simulink model "comparison_simulate_Hinf"  (R2015a)
settings: Solver=ode14x  StartTime=0.0  StopTime=10  FixedStep=1e-4  RelTol=1e-3
values from neighbouring files (symbols this model uses):
  A = [-209.443458109 -450.728478794 0 0 0 0 450.728478794 -209.443458109 0 0 0 0 ... (36 elements, 6x6)]    [comparison.mat]
  AC = [-33660.7984807 29637.8330782 3046.26276086 1989.6816824 595.970985765 1727.63504419 0 0 0 0 0 0 ... (400 elements, 20x20)]    [AC.mat]    (also in h2hinf.m = Kmix.A; hinf.m = K3.A)
  B = [-9.64474367822  2.65660382188; -7.76311006326  -5.61613187293; -0.117927290005  0.0527206875641; 0.215603654719  -0.128623447556; 0.0737096142171  0.0391127484963; -0.0970049785583  -0.0786358112919]    [comparison.mat]
  BC = [23360.0818714 -21011.7426002 -2127.29641138 -1389.45423788 -416.184367151 -1206.45923159 0 0 0 0 0 0 ... (20 elements, 20x1)]    [BC.mat]    (also in h2hinf.m = Kmix.B; hinf.m = K3.B)
  C = [1.88477251669 -1.14284793707 5.77230310808 47.9525873536 -5.11774457916 -49.0010462763]    [comparison.mat]
  CC = [0 0 0 0 0 0 0 0 0 0 0 0 ... (40 elements, 2x20)]    [CC.mat]    (also in h2hinf.m = Kmix.C; hinf.m = K3.C)
  DC = [0 0]    [DC.mat]    (also in h2hinf.m = Kmix.D; hinf.m = K3.D)
  H = [9.64474367822 7.76311006326 0.117927290005 -0.215603654719 -0.0737096142171 0.0970049785583]    [comparison.mat]
  K1 = [2.2796711846  1.62190033935  -10.6282516318  -1.4108556961  -12.4808932363  26.7941597177; 0.146705446363  -9.20812525479  8.2724414747  30.8052765889  17.6744281041  -4.60573511505]    [comparison.mat]
  K2 = [7.68340364795  3.76895934778  4.7809593416  1.0105906737  4.39829283468  -9.14553212992; -11.324326837  11.7994850376  -4.15081128654  -16.3715631545  -6.63659637257  1.48616499821]    [comparison.mat]
  L1 = [25.9427258674 3.21915313057 0.189903086471 -0.425157992773 0.204783234732 0.30836256894]    [comparison.mat]
  L2 = [-17.8178024007 12.2869558648 -0.241266463594 0.355791079936 -0.00240455397922 -0.130577661056]    [comparison.mat]
settings Model: Creator=p4wp4w  LastModifiedBy=p4wp4w

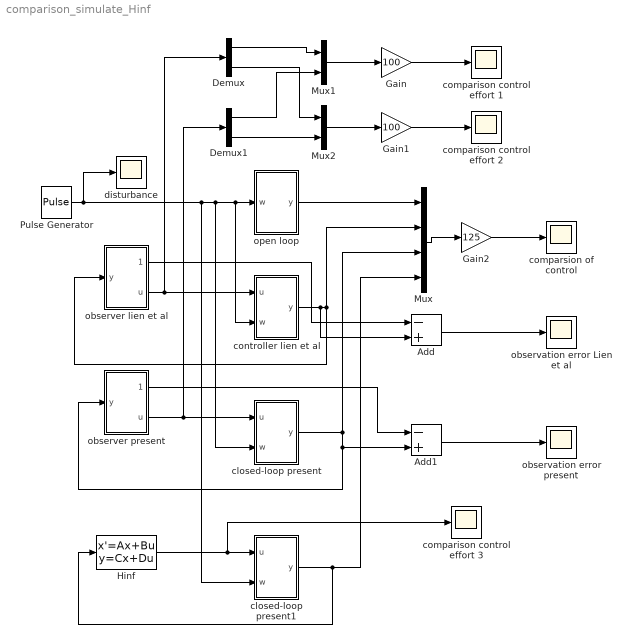
== system comparison_simulate_Hinf ==
  Add : Sum  Inputs=-+
  Add1 : Sum  Inputs=-+
  Demux : Demux  Outputs=2
  Demux1 : Demux  Outputs=2
  Gain : Gain  Gain=100
  Gain1 : Gain  Gain=100
  Gain2 : Gain  Gain=125
  Hinf : StateSpace  A=AC  B=BC  C=CC  D=DC  X0=0
  Mux : Mux
  Mux1 : Mux  Inputs=2
  Mux2 : Mux  Inputs=2
  Pulse Generator : DiscretePulseGenerator  PulseType=Time based  Amplitude=10  Period=5  PulseWidth=50
  closed-loop present : Subsystem
  closed-loop present1 : Subsystem
  comparison control effort 1 : Scope
      settings: SaveName=effort1
  comparison control effort 2 : Scope
      settings: SaveName=effort2
  comparison control effort 3 : Scope
      settings: SaveName=effort
  comparsion of control : Scope
      settings: YMin=-100  YMax=75  SaveName=controlleduncontrolled
  controller lien et al : Subsystem
  disturbance : Scope
      settings: SaveName=disturbance
  observation error Lien et al : Scope
      settings: SaveName=observation_error_Lien
  observation error present : Scope
      settings: SaveName=observation_error_present
  observer lien et al : Subsystem
  observer present : Subsystem
  open loop : Subsystem
  wires:
  controller lien et al/1(y) -> Add/2, Mux/2, observer lien et al/1(y)
  observer lien et al/2(u) -> Demux/1, controller lien et al/1(u)
  Pulse Generator/1 -> disturbance/1, closed-loop present1/2(w), closed-loop present/2(w), controller lien et al/2(w), open loop/1(w)
  observer present/2(u) -> Demux1/1, closed-loop present/1(u)
  closed-loop present/1(y) -> Add1/2, observer present/1(y), Mux/3
  open loop/1(y) -> Mux/1
  Mux/1 -> Gain2/1
  observer lien et al/1(yhat) -> Add/1
  observer present/1(yhat) -> Add1/1
  Mux1/1 -> Gain/1
  Gain/1 -> comparison control effort 1/1
  Mux2/1 -> Gain1/1
  Gain1/1 -> comparison control effort 2/1
  Demux1/1 -> Mux1/2
  Demux/1 -> Mux1/1
  Demux/2 -> Mux2/1
  Demux1/2 -> Mux2/2
  Gain2/1 -> comparsion of control/1
  Add/1 -> observation error Lien et al/1
  Add1/1 -> observation error present/1
  Hinf/1 -> comparison control effort 3/1, closed-loop present1/1(u)
  closed-loop present1/1(y) -> Mux/4, Hinf/1

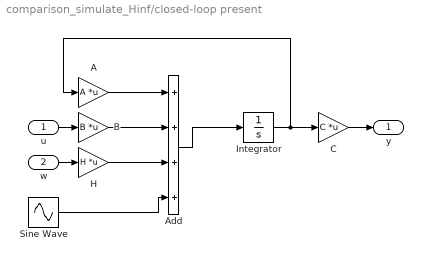
== system comparison_simulate_Hinf/closed-loop present ==
  u : Inport
  w : Inport  Port=2
  A : Gain  Gain=A  Multiplication=Matrix(K*u)
  Add : Sum  Inputs=++++
  B : Gain  Gain=B  Multiplication=Matrix(K*u)
  C : Gain  Gain=C  Multiplication=Matrix(K*u)
  H : Gain  Gain=H  Multiplication=Matrix(K*u)
  Integrator : Integrator
  Sine Wave : Sin  Amplitude=0.01  Frequency=14  SampleTime=0
  y : Outport
  wires:
  C/1 -> y/1
  u/1 -> B/1
  w/1 -> H/1
  H/1 -> Add/3
  Integrator/1 -> A/1, C/1
  A/1 -> Add/1
  B/1 -> Add/2
  Add/1 -> Integrator/1
  Sine Wave/1 -> Add/4

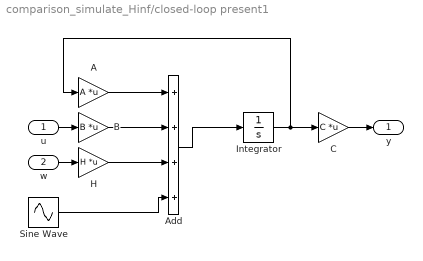
== system comparison_simulate_Hinf/closed-loop present1 ==
  u : Inport
  w : Inport  Port=2
  A : Gain  Gain=A  Multiplication=Matrix(K*u)
  Add : Sum  Inputs=++++
  B : Gain  Gain=B  Multiplication=Matrix(K*u)
  C : Gain  Gain=C  Multiplication=Matrix(K*u)
  H : Gain  Gain=H  Multiplication=Matrix(K*u)
  Integrator : Integrator
  Sine Wave : Sin  Amplitude=0.01  Frequency=14  SampleTime=0
  y : Outport
  wires:
  Sine Wave/1 -> Add/4
  Add/1 -> Integrator/1
  B/1 -> Add/2
  A/1 -> Add/1
  Integrator/1 -> C/1, A/1
  H/1 -> Add/3
  w/1 -> H/1
  u/1 -> B/1
  C/1 -> y/1

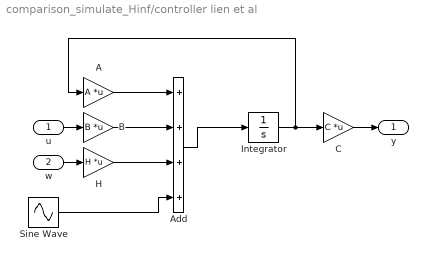
== system comparison_simulate_Hinf/controller lien et al ==
  u : Inport
  w : Inport  Port=2
  A : Gain  Gain=A  Multiplication=Matrix(K*u)
  Add : Sum  Inputs=++++
  B : Gain  Gain=B  Multiplication=Matrix(K*u)
  C : Gain  Gain=C  Multiplication=Matrix(K*u)
  H : Gain  Gain=H  Multiplication=Matrix(K*u)
  Integrator : Integrator
  Sine Wave : Sin  Amplitude=0.01  Frequency=14  SampleTime=0
  y : Outport
  wires:
  Add/1 -> Integrator/1
  B/1 -> Add/2
  A/1 -> Add/1
  Integrator/1 -> C/1, A/1
  H/1 -> Add/3
  w/1 -> H/1
  u/1 -> B/1
  C/1 -> y/1
  Sine Wave/1 -> Add/4

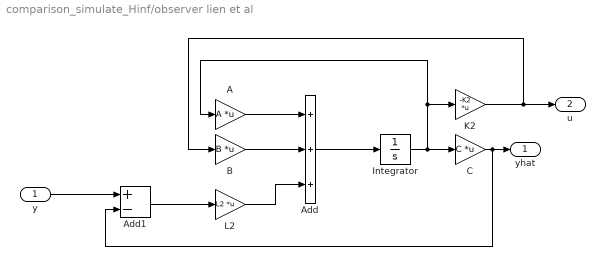
== system comparison_simulate_Hinf/observer lien et al ==
  y : Inport
  A : Gain  Gain=A  Multiplication=Matrix(K*u)
  Add : Sum  Inputs=+++
  Add1 : Sum  Inputs=+-
  B : Gain  Gain=B  Multiplication=Matrix(K*u)
  C : Gain  Gain=C  Multiplication=Matrix(K*u)
  Integrator : Integrator
  K2 : Gain  Gain=-K2  Multiplication=Matrix(K*u)
  L2 : Gain  Gain=L2  Multiplication=Matrix(K*u)
  yhat : Outport
  u : Outport  Port=2
  wires:
  C/1 -> Add1/2, yhat/1
  K2/1 -> B/1, u/1
  Integrator/1 -> K2/1, A/1, C/1
  A/1 -> Add/1
  B/1 -> Add/2
  Add/1 -> Integrator/1
  L2/1 -> Add/3
  Add1/1 -> L2/1
  y/1 -> Add1/1

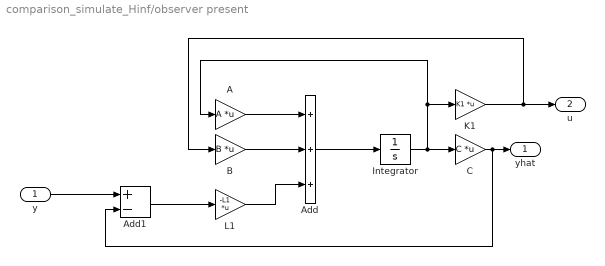
== system comparison_simulate_Hinf/observer present ==
  y : Inport
  A : Gain  Gain=A  Multiplication=Matrix(K*u)
  Add : Sum  Inputs=+++
  Add1 : Sum  Inputs=+-
  B : Gain  Gain=B  Multiplication=Matrix(K*u)
  C : Gain  Gain=C  Multiplication=Matrix(K*u)
  Integrator : Integrator
  K1 : Gain  Gain=K1  Multiplication=Matrix(K*u)
  L1 : Gain  Gain=-L1  Multiplication=Matrix(K*u)
  yhat : Outport
  u : Outport  Port=2
  wires:
  y/1 -> Add1/1
  Add1/1 -> L1/1
  L1/1 -> Add/3
  Add/1 -> Integrator/1
  B/1 -> Add/2
  A/1 -> Add/1
  Integrator/1 -> C/1, A/1, K1/1
  K1/1 -> u/1, B/1
  C/1 -> yhat/1, Add1/2

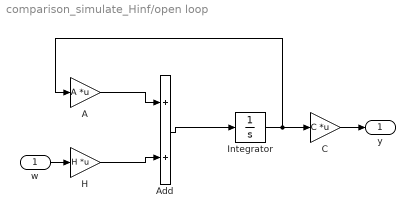
== system comparison_simulate_Hinf/open loop ==
  w : Inport
  A : Gain  Gain=A  Multiplication=Matrix(K*u)
  Add : Sum
  C : Gain  Gain=C  Multiplication=Matrix(K*u)
  H : Gain  Gain=H  Multiplication=Matrix(K*u)
  Integrator : Integrator
  y : Outport
  wires:
  C/1 -> y/1
  w/1 -> H/1
  H/1 -> Add/2
  Integrator/1 -> A/1, C/1
  A/1 -> Add/1
  Add/1 -> Integrator/1
